simulink model "ABS_mpccontroller"  (R2015b)
settings: Solver=ode45  StartTime=0.0  StopTime=30  FixedStep=0.001  RelTol=1e-3
PostLoadFcn:
  | , if any(exist('dsrtsu_mdlpostloadfcn', 'file') == [2, 3, 6]), try dsrtsu_mdlpostloadfcn('Execute', bdroot); catch fprintf('Error in PostLoadFcn (dsrtsu_mdlpostloadfcn) for model "%s":\n %s\n', bdroot, lasterr); end, end,
values from neighbouring files (symbols this model uses):
  A = [-a/v  1/v 0 ... (first row only)    [ABS_mpcdesign.m]    (also in mpc_ssMatrix.m = [0.299843671875         0)
  B = [R/J 0 ... (first row only)    [ABS_mpcdesign.m]    (also in mpc_ssMatrix.m = [0.010667   0.010667)
  C = [0     0    k_reifen ... (first row only)    [ABS_mpcdesign.m]    (also in mpc_ssMatrix.m = [1           0)
  D = [0 0 ... (first row only)    [ABS_mpcdesign.m]    (also in mpc_ssMatrix.m = zeros(2,2))
  T_sollrb = 100    [ABS_mpcdesign.m]
  Td = 1500    [ABS_mpcdesign.m]    (also in ABS_mpcfahrzeugpara.m; Fahrzeug_Parameter.m)
libraries: mpclib x1
settings Model: DSRTSU_INTERNAL_RTI_VER=470  DSRTSU_INTERNAL_RTI_TYPE=rti1401  DSRTSU_INTERNAL_RTIFPGA=60  Creator=MSI  LastModifiedBy=MSI
settings DataIOCC: SaveFormat=Array  SignalLoggingName=sigsOut
settings OptimizationCC: BlockReduction=off
settings DebuggingCC: SaveWithParameterizedLinksMsg=none  UnderspecifiedInitializationDetection=Classic  CheckExecutionContextPreStartOutputMsg=on  CheckExecutionContextRuntimeOutputMsg=on  SignalResolutionControl=TryResolveAllWithWarning  MultiTaskDSMMsg=warning  MultiTaskCondExecSysMsg=none  IntegerOverflowMsg=none  StateNameClashWarn=warning  IntegerSaturationMsg=none
settings HardwareCC: ProdBitPerPointer=32  ProdLargestAtomicInteger=Integer  ProdEndianess=BigEndian  ProdWordSize=32  ProdHWDeviceType=Custom Processor->Custom  TargetIntDivRoundTo=Zero  TargetEndianess=BigEndian  TargetHWDeviceType=Custom Processor->Custom
settings RTWCC: SystemTargetFile=rti1401.tlc  MakeCommand=make_rti  TemplateMakefile=rti1401.tmf  Description=dSPACE DS1401 Hardware Platform
settings STFCustomTargetCC: ParMdlRefBuildCompliant=on  ConcurrentExecutionCompliant=off  GeneratePreprocessorConditionals=Use local settings  MatFileLogging=on  CPPClassGenCompliant=off  SystemTargetFile=rti1401.tlc
settings GRTTargetCC: CompOptLevelCompliant=off  ConcurrentExecutionCompliant=off  CombineOutputUpdateFcns=off  CPPClassGenCompliant=off  GRTInterface=on  UseToolchainInfoCompliant=off  ExtModeMexFile=noextcomm

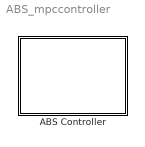
== system ABS_mpccontroller ==
  ABS Controller : Subsystem

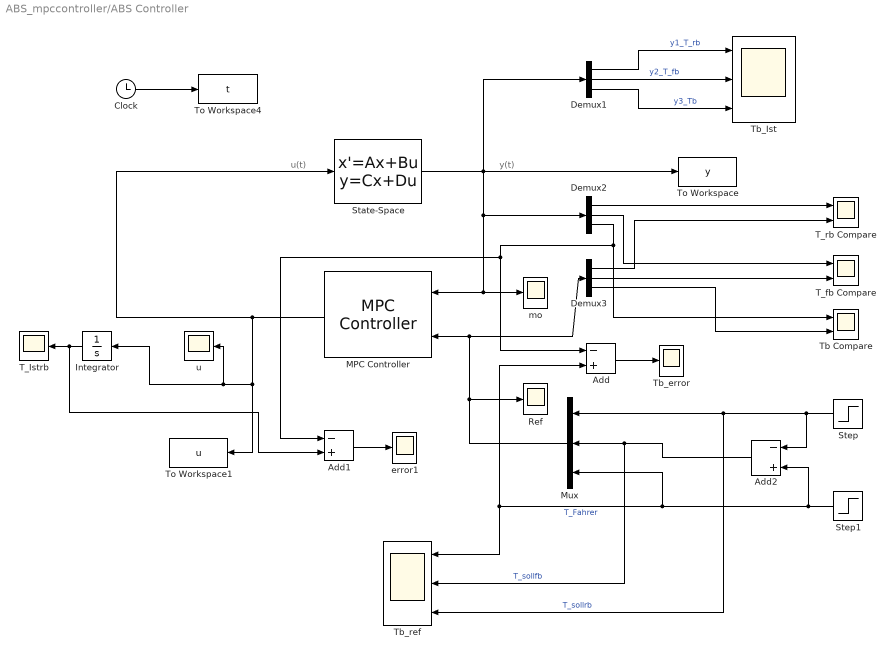
== system ABS_mpccontroller/ABS Controller ==
  note: u(t)
  note: y(t)
  Add : Sum  Inputs=-+
  Add1 : Sum  Inputs=-+
  Add2 : Sum  Inputs=-+
  Clock : Clock
  Demux1 : Demux  Outputs=3
  Demux2 : Demux  Outputs=3
  Demux3 : Demux  Outputs=3
  Integrator : Integrator
  MPC Controller : mpclib/MPC Controller  mpcobj=mpcobj  x0=[]  is_multiple=0  enable_value=0  return_u0=off  ref_from_ws=off  ref_signal_name=[]  ref_preview=on  md_from_ws=off  md_signal_name=[]  md_preview=on  from_project=off  project_file=MPCtask.mat  md_inport=off  mv_inport=off  cost_outport=off  return_sequence=off  return_qpstatus=off  return_state=off  state_inport=off  lims_inport=off  ywt_inport=off  is_designfromscratch=0  uwt_inport=off  duwt_inport=off  rhoeps_inport=off  uref_inport=off  n_ts=0.1  n_mv=2  n_md=0  n_ud=0  n_mo=3  n_uo=0  BlockDataType=double  SampleTimeInherited=off  switch_inport=off
  Mux : Mux  Inputs=3
  Ref : Scope
  State-Space : StateSpace  A=A  B=B  C=C  D=D  X0=0
  Step : Step  After=T_sollrb  SampleTime=0
  Step1 : Step  After=Td  SampleTime=0
  T_Istrb : Scope
  T_fb Compare : Scope  NumInputPorts=2
  T_rb Compare : Scope  NumInputPorts=2
  Tb Compare : Scope  NumInputPorts=2
  Tb_Ist : Scope  NumInputPorts=3
  Tb_error : Scope
  Tb_ref : Scope  NumInputPorts=3
  To Workspace : ToWorkspace  VariableName=y  SampleTime=-1
      settings: MaxDataPoints=Inf
  To Workspace1 : ToWorkspace  VariableName=u  SampleTime=-1
      settings: MaxDataPoints=Inf
  To Workspace4 : ToWorkspace  VariableName=t  SampleTime=-1
      settings: MaxDataPoints=Inf
  error1 : Scope
  mo : Scope
  u : Scope
  wires:
  State-Space/1 -> Demux1/1, To Workspace/1, Demux2/1, MPC Controller/1, mo/1
  Add/1 -> Tb_error/1
  Step1/1 -> Add2/2, Mux/3, Add/2, Tb_ref/1  "T_Fahrer"
  MPC Controller/1 -> u/1, Integrator/1, To Workspace1/1, State-Space/1
  Clock/1 -> To Workspace4/1
  Integrator/1 -> Add1/2, T_Istrb/1
  Add1/1 -> error1/1
  Step/1 -> Tb_ref/3, Mux/1, Add2/1  "T_sollrb"
  Add2/1 -> Tb_ref/2, Mux/2  "T_sollfb"
  Mux/1 -> Ref/1, Demux3/1, MPC Controller/2
  Demux1/1 -> Tb_Ist/1  "y1_T_rb"
  Demux1/2 -> Tb_Ist/2  "y2_T_fb"
  Demux1/3 -> Tb_Ist/3  "y3_Tb"
  Demux2/1 -> T_rb Compare/1
  Demux2/2 -> T_fb Compare/1
  Demux2/3 -> Add1/1, Add/1, Tb Compare/1
  Demux3/1 -> T_rb Compare/2
  Demux3/2 -> T_fb Compare/2
  Demux3/3 -> Tb Compare/2
